simulink library "Subchart_Step_Response"  (R2022b)
settings: Solver=VariableStepAuto  StartTime=0.0  StopTime=10.0  RelTol=1e-3
settings Model: Creator=valen  LastModifiedBy=valen
settings DebuggingCC: UnconnectedInputMsg=warning  UnconnectedOutputMsg=warning  UnconnectedLineMsg=warning
settings ModelReferenceCC: EnableRefExpFcnMdlSchedulingChecks=on
settings RTWCC: DLArmComputeVersion=19.05

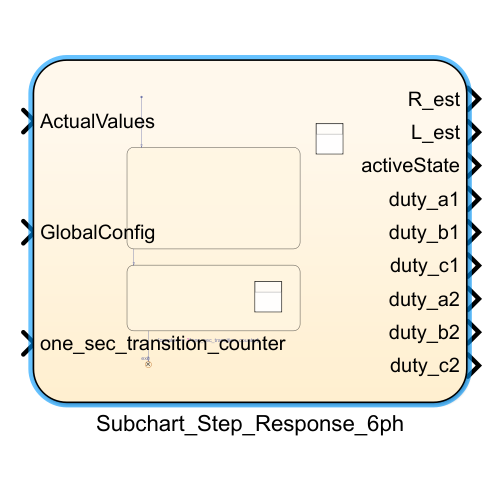
[thumbnail: Simulink's stored preview of the top-level diagram]
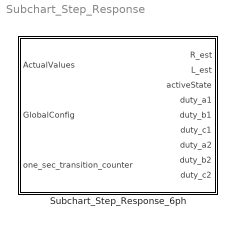
== system Subchart_Step_Response ==
  Subchart_Step_Response_6ph : Stateflow chart  TreatAsAtomicUnit=on

== stateflow chart Subchart_Step_Response/Subchart_Step_Response_6ph ==
  settings: executeAtInitialization=1  initializeOutput=1  description=Dampingfactor
  state stepResponse
    entry:
    activeState = uint16(130)+index;
    setp_dq(index)=ref_amplitude;%setpoints in dq
    setp_abc = inv_VSD*setp_dq;%setpoints in abc
    duty_a1 = GenerateDutyCycle(ActualValues.V_DC, setp_abc(1));
    duty_b1 = GenerateDutyCycle(ActualValues.V_DC, setp_abc(2));
    duty_c1 = GenerateDutyCycle(ActualValues.V_DC, setp_abc(3));
    duty_a2 = GenerateDutyCycle(ActualValues.V_DC, setp_abc(4));
    duty_b2 = GenerateDutyCycle(ActualValues.V_DC, setp_abc(5));
    duty_c2 = GenerateDutyCycle(ActualValues.V_DC, setp_abc(6));
    during:
    MeasureStepResponse(ActualValues.v_dq_6ph,ActualValues.i_dq_6ph);
    counter = counter +1;
    exit:
    duty_a1 = single(0);
    duty_b1 = single(0);
    duty_c1 = single(0);
    duty_a2 = single(0);
    duty_b2 = single(0);
    duty_c2 = single(0);
  state Levenberg_Marquardt
    entry:
    counter = 1;
    LM_algorithm;
    R_est = (R_est-R_corr);
    during:
    counter = counter +1;
    exit:
  (default) -> stepResponse
  stepResponse -> Levenberg_Marquardt : [counter == 1026]
  Levenberg_Marquardt -> 60 : [counter == 3*one_sec_transition_counter]
  data: v_dq function_input Bus: uz_6ph_dq_t size=1; i_dq function_input Bus: uz_6ph_dq_t size=1; setp_abc local single size=[6,1]; setp_dq local single size=[6,1]; k local single size=1 =single(0); dp local single size=[2,1] =single(0); e local single size=1 =single(0); e_lm local single size=1 =single(0); it local uint16 size=1 =uint16(0); H local single size=[2,2] =single(0); L0 local single size=1 =single(0); R0 local single size=1 =single(0); n_iters local uint16 size=1 =uint16(100); lambda local single size=1 =single(0.01); updateJ local boolean size=1 =true; d local single size=[2048,1] =single(0); i_est local single size=[2048,1] =single(0); J local single size=[2048,2] =single(0); R_lm local single size=1 =single(0); L_lm local single size=1 =single(0); R_corr local single size=1 =single(0); counter local uint32 size=1 =uint32(1); ActualValues input Bus: uz_ParaID_ActualValues_t; GlobalConfig input Bus: uz_ParaID_GlobalConfig_t size=1; Vstep local single size=[205,1] =single(0); ref_amplitude data_store_memory size=1; inv_VSD constant single size=[6,6] =inv_VSD; current_meas_array local single size=[1024,1] =single(0); index parameter uint16 size=1 [uint16(1)..uint16(5)]; R_est output single size=1 =single(0); L_est output single size=1 =single(0); z local uint16 size=1 =uint16(1); V0 local single size=1 =single(0); activeState output uint16 size=1 =uint16(0); one_sec_transition_counter input uint32 size=1; voltage_meas_array local single size=[1024,1] =single(0); duty_a1 output single size=1; duty_b1 output single size=1; duty_c1 output single size=1; duty_a2 output single size=1; duty_b2 output single size=1; duty_c2 output single size=1
  data k settings: description=counting variable (for loop)
  data dp settings: description=new parameter estimation
  data e settings: description=Error squared
  data e_lm settings: description=updated quared error
  data it settings: description=current iteration
  data H settings: description=Hesse Matrix
  data L0 settings: description=start value
  data R0 settings: description=start value
  data n_iters settings: description=number of iterations
  data lambda settings: description=Dampingfactor
  data updateJ settings: description=Flag: update Jakobinian matrix or not
  data d settings: description=error meas data and approx data
  data i_est settings: description=calculated current step response for estimated parameters
  data J settings: description=Jacobian matrix
  data R_lm settings: description=updated parameter estimation
  data L_lm settings: description=updated parameter estimation
  data counter settings: description=couting variable
  data Vstep settings: description=record of voltage step
  data ref_amplitude settings: description=Reference amplitude
  data z settings: description=counting varialble for voltage step recording
  data V0 settings: description=medium voltage
  function MeasureStepResponse(v_dq,i_dq):
    | function MeasureStepResponse(v_dq,i_dq)
    | fns = fieldnames(i_dq);
    | current = i_dq.(fns{index});
    | voltage = v_dq.(fns{index});
    | if(counter <= 1024)
    |     if(counter > 1)
    |         current_meas_array(counter-1) = current;%safe 1024 current values to 2D array
    |         voltage_meas_array(counter-1) = voltage;
    |         if(mod(counter,5) == 0)%exec every 5th cycle
    |             Vstep(z-1) = voltage;%safe Va
    |             z = z + 1;
    |         end
    |     elseif(counter == 1)
    |         Vstep(1) = voltage;%safe Va 1st cycle
    |         z = z + 1;
    |     end
    | else
    |     if(counter == 1025)
    |         current_meas_array(counter-1) = current;%safe last current val
    |         voltage_meas_array(counter-1) = voltage;
    |         Vstep(z-1) = voltage;
    |         V0 = mean(voltage_meas_array);%average voltage
    |     end
    | end
    | end
  function LM_algorithm:
    | function LM_algorithm
    |    
    |     
    | % Startwerte Festlegen
    | %V0 = V_s;                           % Spannungssprung in Volt
    | R0 = single(0.001000);              % Widerstand in Ohm (0.01 ... 40 Ohm)
    | L0 = single(0.000005);              % Induktivitaet in Henry (0.05mH ... 50 mH)
    | 
    | R_est   = R0;
    | L_est   = L0;
    | %#codegen
    | 
    | % Levenberg-Marquardt Curve Fitting
    | 
    | % i_input(Stromwerte) -> Stromwerte in A !!!
    | 
    | % Mathematische Grundlagen mit Symbolic Toolbox erstellen
    |     %syms U R L t i real;                   %Symbolische Variablen erstellen
    |     %f = U/R*(1-exp(-R*t/L))                %Modellfunktion (Laden einer Spule)
    |     %d = i-f;                               %Fehler d = Messung - Modell
    |     %Jsym = jacobian(d,[R L])               %Jacobi-Matrix des Fehlers (Ableitungen nach den Parametern R und L)                  
    | 
    |     
    |     % Parameterbestimmung durch Iteration
    |     for it=uint16(1):n_iters
    |         if updateJ == 1
    |             % Jacobi-Matrix mit aktuellem Parametersatz berechnen
    |             for k=single(1):single(1024)
    |              J(k,:) = [- (V0*(exp(-(R_est*(k-1)*GlobalConfig.sampleTimeISR)/L_est)....
    |                  - 1))/R_est^2 - (V0*(k-1)*GlobalConfig.sampleTimeISR*exp....
    |                  (-(R_est*(k-1)*GlobalConfig.sampleTimeISR)/L_est))/(L_est*R_est)....
    |                  , (V0*(k-1)*GlobalConfig.sampleTimeISR*exp(-(R_est*(k-1)*....
    |                  GlobalConfig.sampleTimeISR)/L_est))/L_est^2];
    |             end
    |             % Modellfunktion mit aktuellem Parametersatz berechnen
    |             for k=single(1):single(1024)
    |             i_est(k) = V0/R_est*(1-exp(-R_est*((k-1)*GlobalConfig.sampleTimeISR)/L_est));
    |             end
    |             % Fehler zwischen Messdaten und Modellfunktionswerten berechnen
    |             d(1:1024) = current_meas_array(1:1024)-i_est(1:1024);
    |             % Approximierte Hesse-Matrix berechnen
    |             H = J(1:1024,:)'*J(1:1024,:);
    |             if it==1
    |                 e = dot(d,d);           % Fehlerquadrat berechnen
    |             end
    |         end
    |         
    |         % Daempfungsfaktor lambda auf Hesse-Matrix anwenden
    |         H(1,1) = H(1,1) + lambda;
    |         H(2,2)=H(2,2)+lambda;
    |         
    |         % Neue Paramterschaetzung berechnen
    |         dp = -inv(H)*(J(1:1024,:)'*d(1:1024));
    |         R_lm = R_est + dp(1);
    |         L_lm = L_est + dp(2);
    |         
    |         % Modellfunktion mit neuem Parametersatz berechnen
    |         for k=single(1):single(1024)
    |         i_est(k) = V0/R_lm*(1-exp(-R_lm*((k-1)*GlobalConfig.sampleTimeISR)/L_lm));
    |         end
    |         % Fehler und Fehlerquadrate neu berechnen
    |         d(1:1024) = current_meas_array(1:1024) - i_est(1:1024);
    |         e_lm = dot(d(1:1024),d(1:1024));
    |         
    |         % Fallunterscheidung ob Fehler groesser oder kleiner geworden ist
    |         if e_lm < e
    |             lambda = lambda/10;
    |             R_est = R_lm;
    |             L_est = L_lm;
    |             e = e_lm;
    |             updateJ = boolean(1);
    |         else
    |             updateJ = boolean(0);
    |             lambda = lambda*10;
    |         end
    |     end
